simulink model "Pendolo_Inverso"  (R2019b)
(part 3 of 12)

  Transform/LConn1 -- ReferenceFrame/RConn1 -- Transform1/LConn1 -- Transform10/LConn1 -- Transform100/LConn1 -- Transform101/LConn1 -- Transform102/LConn1 -- Transform103/LConn1 -- Transform104/LConn1 -- Transform105/LConn1 -- Transform106/LConn1 -- Transform107/LConn1 -- Transform108/LConn1 -- Transform109/LConn1 -- Transform11/LConn1 -- Transform110/LConn1 -- Transform111/LConn1 -- Transform112/LConn1 -- Transform113/LConn1 -- Transform114/LConn1 -- Transform115/LConn1 -- Transform116/LConn1 -- Transform117/LConn1 -- Transform118/LConn1 -- Transform119/LConn1 -- Transform12/LConn1 -- Transform120/LConn1 -- Transform121/LConn1 -- Transform122/LConn1 -- Transform123/LConn1 -- Transform124/LConn1 -- Transform125/LConn1 -- Transform126/LConn1 -- Transform127/LConn1 -- Transform128/LConn1 -- Transform129/LConn1 -- Transform13/LConn1 -- Transform130/LConn1 -- Transform131/LConn1 -- Transform132/LConn1 -- Transform133/LConn1 -- Transform134/LConn1 -- Transform135/LConn1 -- Transform136/LConn1 -- Transform137/LConn1 -- Transform138/LConn1 -- Transform139/LConn1 -- Transform14/LConn1 -- Transform140/LConn1 -- Transform141/LConn1 -- Transform142/LConn1 -- Transform143/LConn1 -- Transform144/LConn1 -- Transform145/LConn1 -- Transform146/LConn1 -- Transform147/LConn1 -- Transform148/LConn1 -- Transform149/LConn1 -- Transform15/LConn1 -- Transform150/LConn1 -- Transform151/LConn1 -- Transform152/LConn1 -- Transform153/LConn1 -- Transform154/LConn1 -- Transform155/LConn1 -- Transform156/LConn1 -- Transform157/LConn1 -- Transform158/LConn1 -- Transform159/LConn1 -- Transform16/LConn1 -- Transform160/LConn1 -- Transform17/LConn1 -- Transform18/LConn1 -- Transform19/LConn1 -- Transform2/LConn1 -- Transform20/LConn1 -- Transform21/LConn1 -- Transform22/LConn1 -- Transform23/LConn1 -- Transform24/LConn1 -- Transform25/LConn1 -- Transform26/LConn1 -- Transform27/LConn1 -- Transform28/LConn1 -- Transform29/LConn1 -- Transform3/LConn1 -- Transform30/LConn1 -- Transform31/LConn1 -- Transform32/LConn1 -- Transform33/LConn1 -- Transform34/LConn1 -- Transform35/LConn1 -- Transform36/LConn1 -- Transform37/LConn1 -- Transform38/LConn1 -- Transform39/LConn1 -- Transform4/LConn1 -- Transform40/LConn1 -- Transform41/LConn1 -- Transform42/LConn1 -- Transform43/LConn1 -- Transform44/LConn1 -- Transform45/LConn1 -- Transform46/LConn1 -- Transform47/LConn1 -- Transform48/LConn1 -- Transform49/LConn1 -- Transform5/LConn1 -- Transform50/LConn1 -- Transform51/LConn1 -- Transform52/LConn1 -- Transform53/LConn1 -- Transform54/LConn1 -- Transform55/LConn1 -- Transform56/LConn1 -- Transform57/LConn1 -- Transform58/LConn1 -- Transform59/LConn1 -- Transform6/LConn1 -- Transform60/LConn1 -- Transform61/LConn1 -- Transform62/LConn1 -- Transform63/LConn1 -- Transform64/LConn1 -- Transform65/LConn1 -- Transform66/LConn1 -- Transform67/LConn1 -- Transform68/LConn1 -- Transform69/LConn1 -- Transform7/LConn1 -- Transform70/LConn1 -- Transform71/LConn1 -- Transform72/LConn1 -- Transform73/LConn1 -- Transform74/LConn1 -- Transform75/LConn1 -- Transform76/LConn1 -- Transform77/LConn1 -- Transform78/LConn1 -- Transform79/LConn1 -- Transform8/LConn1 -- Transform80/LConn1 -- Transform81/LConn1 -- Transform82/LConn1 -- Transform83/LConn1 -- Transform84/LConn1 -- Transform85/LConn1 -- Transform86/LConn1 -- Transform87/LConn1 -- Transform88/LConn1 -- Transform89/LConn1 -- Transform9/LConn1 -- Transform90/LConn1 -- Transform91/LConn1 -- Transform92/LConn1 -- Transform93/LConn1 -- Transform94/LConn1 -- Transform95/LConn1 -- Transform96/LConn1 -- Transform97/LConn1 -- Transform98/LConn1 -- Transform99/LConn1
  Transform/RConn1 -- F/RConn1
  Transform9/RConn1 -- x28_Rondella_M63_RIGID/LConn1
  Transform99/RConn1 -- x28_Rondella_M663_RIGID/LConn1
  Transform100/RConn1 -- x28_Rondella_M664_RIGID/LConn1
  Transform101/RConn1 -- x28_Rondella_M665_RIGID/LConn1
  Transform102/RConn1 -- x28_Rondella_M666_RIGID/LConn1
  DIN_1587_M612_RIGID/LConn1 -- Transform103/RConn1
  DIN_934_sostituito_da_DIN_EN_24032_28673_28674_M612_RIGID/LConn1 -- Transform104/RConn1
  Transform105/RConn1 -- x28_Rondella_M667_RIGID/LConn1
  DIN_933_sostituito_da_DIN_EN_24017_M6_x_3012_RIGID/LConn1 -- Transform106/RConn1
  Transform107/RConn1 -- x28_Rondella_M668_RIGID/LConn1
  Transform108/RConn1 -- x28_Rondella_M669_RIGID/LConn1
  Transform10/RConn1 -- x28_Rondella_M64_RIGID/LConn1
  Transform109/RConn1 -- x28_Rondella_M670_RIGID/LConn1
  Transform110/RConn1 -- x28_Rondella_M671_RIGID/LConn1
  Transform111/RConn1 -- x28_Rondella_M672_RIGID/LConn1
  DIN_1587_M613_RIGID/LConn1 -- Transform112/RConn1
  DIN_934_sostituito_da_DIN_EN_24032_28673_28674_M613_RIGID/LConn1 -- Transform113/RConn1
  Transform114/RConn1 -- x28_Rondella_M673_RIGID/LConn1
  DIN_933_sostituito_da_DIN_EN_24017_M6_x_3013_RIGID/LConn1 -- Transform115/RConn1
  Transform116/RConn1 -- x28_Rondella_M674_RIGID/LConn1
  Transform117/RConn1 -- x28_Rondella_M675_RIGID/LConn1
  Transform118/RConn1 -- x28_Rondella_M676_RIGID/LConn1
  Transform11/RConn1 -- x28_Rondella_M65_RIGID/LConn1
  Transform119/RConn1 -- x28_Rondella_M677_RIGID/LConn1
  Transform120/RConn1 -- x28_Rondella_M678_RIGID/LConn1
  DIN_1587_M614_RIGID/LConn1 -- Transform121/RConn1
  DIN_934_sostituito_da_DIN_EN_24032_28673_28674_M614_RIGID/LConn1 -- Transform122/RConn1
  Transform123/RConn1 -- x28_Rondella_M679_RIGID/LConn1
  DIN_933_sostituito_da_DIN_EN_24017_M6_x_3014_RIGID/LConn1 -- Transform124/RConn1
  Transform125/RConn1 -- x28_Rondella_M680_RIGID/LConn1
  Transform126/RConn1 -- x28_Rondella_M681_RIGID/LConn1
  Transform127/RConn1 -- x28_Rondella_M682_RIGID/LConn1
  Transform128/RConn1 -- x28_Rondella_M683_RIGID/LConn1
  Transform12/RConn1 -- x28_Rondella_M66_RIGID/LConn1
  Transform129/RConn1 -- x28_Rondella_M684_RIGID/LConn1
  DIN_1587_M615_RIGID/LConn1 -- Transform130/RConn1
  DIN_934_sostituito_da_DIN_EN_24032_28673_28674_M615_RIGID/LConn1 -- Transform131/RConn1
  Transform132/RConn1 -- x28_Rondella_M685_RIGID/LConn1
  DIN_933_sostituito_da_DIN_EN_24017_M6_x_3015_RIGID/LConn1 -- Transform133/RConn1
  Transform134/RConn1 -- x28_Rondella_M686_RIGID/LConn1
  Transform135/RConn1 -- x28_Rondella_M687_RIGID/LConn1
  Transform136/RConn1 -- x28_Rondella_M688_RIGID/LConn1
  Transform137/RConn1 -- x28_Rondella_M689_RIGID/LConn1
  Transform138/RConn1 -- x28_Rondella_M690_RIGID/LConn1
  DIN_1587_M62_RIGID/LConn1 -- Transform13/RConn1
  DIN_1587_M616_RIGID/LConn1 -- Transform139/RConn1
  DIN_934_sostituito_da_DIN_EN_24032_28673_28674_M616_RIGID/LConn1 -- Transform140/RConn1
  Transform141/RConn1 -- x28_Rondella_M691_RIGID/LConn1
  DIN_933_sostituito_da_DIN_EN_24017_M6_x_3016_RIGID/LConn1 -- Transform142/RConn1
  Transform143/RConn1 -- x28_Rondella_M692_RIGID/LConn1
  Transform144/RConn1 -- x28_Rondella_M693_RIGID/LConn1
  Transform145/RConn1 -- x28_Rondella_M694_RIGID/LConn1
  Transform146/RConn1 -- x28_Rondella_M695_RIGID/LConn1
  Transform147/RConn1 -- x28_Rondella_M696_RIGID/LConn1
  Transform148/RConn1 -- x26_Collana_di_Sfere1_RIGID/LConn1
  DIN_934_sostituito_da_DIN_EN_24032_28673_28674_M62_RIGID/LConn1 -- Transform14/RConn1
  AS_1237_2_1_31_RIGID/LConn1 -- Transform149/RConn1
  AS_1110_Metrico_M3_x_251_RIGID/LConn1 -- Transform150/RConn1
  AS_1112_2_Metrico_M3_Tipo_51_RIGID/LConn1 -- Transform151/RConn1
  AS_1110_Metrico_M3_x_252_RIGID/LConn1 -- Transform152/RConn1
  AS_1237_2_1_32_RIGID/LConn1 -- Transform153/RConn1
  AS_1112_2_Metrico_M3_Tipo_52_RIGID/LConn1 -- Transform154/RConn1
  AS_1110_Metrico_M3_x_253_RIGID/LConn1 -- Transform155/RConn1
  AS_1237_2_1_33_RIGID/LConn1 -- Transform156/RConn1
  AS_1112_2_Metrico_M3_Tipo_53_RIGID/LConn1 -- Transform157/RConn1
  AS_1110_Metrico_M3_x_254_RIGID/LConn1 -- Transform158/RConn1
  Transform15/RConn1 -- x28_Rondella_M67_RIGID/LConn1
  AS_1237_2_1_34_RIGID/LConn1 -- Transform159/RConn1
  AS_1112_2_Metrico_M3_Tipo_54_RIGID/LConn1 -- Transform160/RConn1
  DIN_933_sostituito_da_DIN_EN_24017_M6_x_302_RIGID/LConn1 -- Transform16/RConn1
  Transform17/RConn1 -- x28_Rondella_M68_RIGID/LConn1
  Transform18/RConn1 -- x28_Rondella_M69_RIGID/LConn1
  Transform1/RConn1 -- x9_Flangia1_RIGID/LConn1
  Transform19/RConn1 -- x28_Rondella_M610_RIGID/LConn1
  Transform20/RConn1 -- x28_Rondella_M611_RIGID/LConn1
  Transform21/RConn1 -- x28_Rondella_M612_RIGID/LConn1
  DIN_1587_M63_RIGID/LConn1 -- Transform22/RConn1
  DIN_934_sostituito_da_DIN_EN_24032_28673_28674_M63_RIGID/LConn1 -- Transform23/RConn1
  Transform24/RConn1 -- x28_Rondella_M613_RIGID/LConn1
  DIN_933_sostituito_da_DIN_EN_24017_M6_x_303_RIGID/LConn1 -- Transform25/RConn1
  Transform26/RConn1 -- x28_Rondella_M614_RIGID/LConn1
  Transform27/RConn1 -- x28_Rondella_M615_RIGID/LConn1
  Transform28/RConn1 -- x28_Rondella_M616_RIGID/LConn1
  Transform2/RConn1 -- x24_Disco1_RIGID/LConn1
  Transform29/RConn1 -- x28_Rondella_M617_RIGID/LConn1
  Transform30/RConn1 -- x28_Rondella_M618_RIGID/LConn1
  DIN_1587_M64_RIGID/LConn1 -- Transform31/RConn1
  DIN_934_sostituito_da_DIN_EN_24032_28673_28674_M64_RIGID/LConn1 -- Transform32/RConn1
  Transform33/RConn1 -- x28_Rondella_M619_RIGID/LConn1
  DIN_933_sostituito_da_DIN_EN_24017_M6_x_304_RIGID/LConn1 -- Transform34/RConn1
  Transform35/RConn1 -- x28_Rondella_M620_RIGID/LConn1
  Transform36/RConn1 -- x28_Rondella_M621_RIGID/LConn1
  Transform37/RConn1 -- x28_Rondella_M622_RIGID/LConn1
  Transform38/RConn1 -- x28_Rondella_M623_RIGID/LConn1
  Transform3/RConn1 -- x24_Disco2_RIGID/LConn1
  Transform39/RConn1 -- x28_Rondella_M624_RIGID/LConn1
  DIN_1587_M65_RIGID/LConn1 -- Transform40/RConn1
  DIN_934_sostituito_da_DIN_EN_24032_28673_28674_M65_RIGID/LConn1 -- Transform41/RConn1
  Transform42/RConn1 -- x28_Rondella_M625_RIGID/LConn1
  DIN_933_sostituito_da_DIN_EN_24017_M6_x_305_RIGID/LConn1 -- Transform43/RConn1
  Transform44/RConn1 -- x28_Rondella_M626_RIGID/LConn1
  Transform45/RConn1 -- x28_Rondella_M627_RIGID/LConn1
  Transform46/RConn1 -- x28_Rondella_M628_RIGID/LConn1
  Transform47/RConn1 -- x28_Rondella_M629_RIGID/LConn1
  Transform48/RConn1 -- x28_Rondella_M630_RIGID/LConn1
  DIN_1587_M61_RIGID/LConn1 -- Transform4/RConn1
  DIN_1587_M66_RIGID/LConn1 -- Transform49/RConn1
  DIN_934_sostituito_da_DIN_EN_24032_28673_28674_M66_RIGID/LConn1 -- Transform50/RConn1
  Transform51/RConn1 -- x28_Rondella_M631_RIGID/LConn1
  DIN_933_sostituito_da_DIN_EN_24017_M6_x_306_RIGID/LConn1 -- Transform52/RConn1
  Transform53/RConn1 -- x28_Rondella_M632_RIGID/LConn1
  Transform54/RConn1 -- x28_Rondella_M633_RIGID/LConn1
  Transform55/RConn1 -- x28_Rondella_M634_RIGID/LConn1
  Transform56/RConn1 -- x28_Rondella_M635_RIGID/LConn1
  Transform57/RConn1 -- x28_Rondella_M636_RIGID/LConn1
  DIN_1587_M67_RIGID/LConn1 -- Transform58/RConn1
  DIN_934_sostituito_da_DIN_EN_24032_28673_28674_M61_RIGID/LConn1 -- Transform5/RConn1
  DIN_934_sostituito_da_DIN_EN_24032_28673_28674_M67_RIGID/LConn1 -- Transform59/RConn1
  Transform60/RConn1 -- x28_Rondella_M637_RIGID/LConn1
  DIN_933_sostituito_da_DIN_EN_24017_M6_x_307_RIGID/LConn1 -- Transform61/RConn1
  Transform62/RConn1 -- x28_Rondella_M638_RIGID/LConn1
  Transform63/RConn1 -- x28_Rondella_M639_RIGID/LConn1
  Transform64/RConn1 -- x28_Rondella_M640_RIGID/LConn1
  Transform65/RConn1 -- x28_Rondella_M641_RIGID/LConn1
  Transform66/RConn1 -- x28_Rondella_M642_RIGID/LConn1
  DIN_1587_M68_RIGID/LConn1 -- Transform67/RConn1
  DIN_934_sostituito_da_DIN_EN_24032_28673_28674_M68_RIGID/LConn1 -- Transform68/RConn1
  Transform6/RConn1 -- x28_Rondella_M61_RIGID/LConn1
  Transform69/RConn1 -- x28_Rondella_M643_RIGID/LConn1
  DIN_933_sostituito_da_DIN_EN_24017_M6_x_308_RIGID/LConn1 -- Transform70/RConn1
  Transform71/RConn1 -- x28_Rondella_M644_RIGID/LConn1
  Transform72/RConn1 -- x28_Rondella_M645_RIGID/LConn1
  Transform73/RConn1 -- x28_Rondella_M646_RIGID/LConn1
  Transform74/RConn1 -- x28_Rondella_M647_RIGID/LConn1
  Transform75/RConn1 -- x28_Rondella_M648_RIGID/LConn1
  DIN_1587_M69_RIGID/LConn1 -- Transform76/RConn1
  DIN_934_sostituito_da_DIN_EN_24032_28673_28674_M69_RIGID/LConn1 -- Transform77/RConn1
  Transform78/RConn1 -- x28_Rondella_M649_RIGID/LConn1
  DIN_933_sostituito_da_DIN_EN_24017_M6_x_301_RIGID/LConn1 -- Transform7/RConn1
  DIN_933_sostituito_da_DIN_EN_24017_M6_x_309_RIGID/LConn1 -- Transform79/RConn1
  Transform80/RConn1 -- x28_Rondella_M650_RIGID/LConn1
  Transform81/RConn1 -- x28_Rondella_M651_RIGID/LConn1
  Transform82/RConn1 -- x28_Rondella_M652_RIGID/LConn1
  Transform83/RConn1 -- x28_Rondella_M653_RIGID/LConn1
  Transform84/RConn1 -- x28_Rondella_M654_RIGID/LConn1
  DIN_1587_M610_RIGID/LConn1 -- Transform85/RConn1
  DIN_934_sostituito_da_DIN_EN_24032_28673_28674_M610_RIGID/LConn1 -- Transform86/RConn1
  Transform87/RConn1 -- x28_Rondella_M655_RIGID/LConn1
  DIN_933_sostituito_da_DIN_EN_24017_M6_x_3010_RIGID/LConn1 -- Transform88/RConn1
  Transform8/RConn1 -- x28_Rondella_M62_RIGID/LConn1
  Transform89/RConn1 -- x28_Rondella_M656_RIGID/LConn1
  Transform90/RConn1 -- x28_Rondella_M657_RIGID/LConn1
  Transform91/RConn1 -- x28_Rondella_M658_RIGID/LConn1
  Transform92/RConn1 -- x28_Rondella_M659_RIGID/LConn1
  Transform93/RConn1 -- x28_Rondella_M660_RIGID/LConn1
  DIN_1587_M611_RIGID/LConn1 -- Transform94/RConn1
  DIN_934_sostituito_da_DIN_EN_24032_28673_28674_M611_RIGID/LConn1 -- Transform95/RConn1
  Transform96/RConn1 -- x28_Rondella_M661_RIGID/LConn1
  DIN_933_sostituito_da_DIN_EN_24017_M6_x_3011_RIGID/LConn1 -- Transform97/RConn1
  Transform98/RConn1 -- x28_Rondella_M662_RIGID/LConn1
